simulink model "sampleModel1721"  (R2023a)
settings: Solver=VariableStepAuto  StartTime=0.0  StopTime=10.0  RelTol=1e-3
libraries: hdlsllib x3, simulink x1
settings Model: Creator=user1  LastModifiedBy=user1

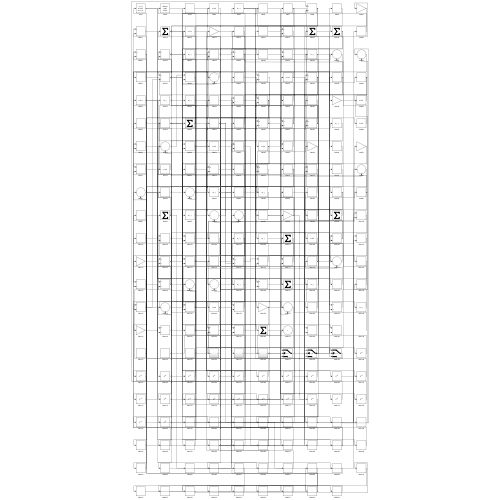
[thumbnail: Simulink's stored preview of the top-level diagram]
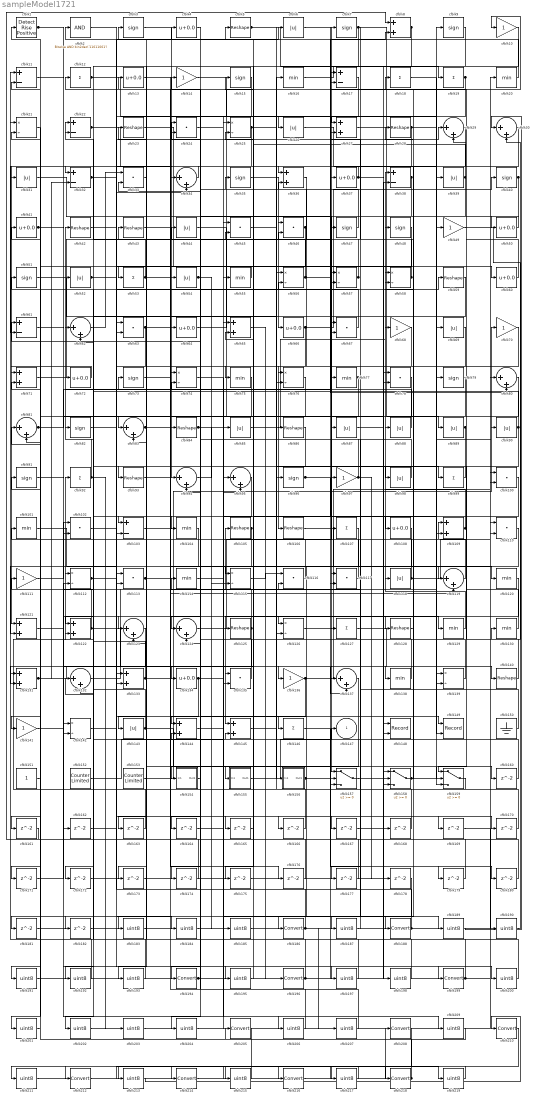
== system sampleModel1721 ==
  cfblk1 : hdlsllib/Logic and Bit Operations/Detect Rise Positive  vinit=0  OutDataTypeStr=boolean
  cfblk{10,14,49,68,70,97,111,136,141} (9 alike) : Gain
  cfblk{24,33,45..46,63,67,78,100,102,110,113,116..117,135} (14 alike) : DotProduct  OutDataTypeStr=Inherit: Inherit via internal rule
  cfblk{16,20,55,75,77,101,104,114,120,129..130,138} (12 alike) : MinMax
  cfblk{11,17,22,32,38,61,103} (7 alike) : Sum  Inputs=+-
  cfblk{5,23,28,42..43,59,84,86,93,105..106,125,128,140} (14 alike) : Reshape
  cfblk{12,18..19,53,92,99,107,127,146} (9 alike) : Sum  Inputs=+
  cfblk{4,13,37,41,50,60,64,66,72,108,134} (11 alike) : Bias  Bias=0.0  SaturateOnIntegerOverflow=off
  cfblk{8,27,36,65,71,109,121..122,131,133,144..145} (12 alike) : Sum
  cfblk{21,25,56..58,74,76,112,115,126,139,142} (12 alike) : Product  Inputs=*/  RndMeth=Zero  SaturateOnIntegerOverflow=on
  cfblk{6,26,31,39,44,52,54,69,85,87..90,98,118,143} (16 alike) : Abs  SaturateOnIntegerOverflow=off
  cfblk{29..30,34,62,80..81,83,94..95,119,123..124,132,137} (14 alike) : Sum  Inputs=|++
  cfblk148 : Record  FileSettingsInternal="{\"entries\":[{\"content\":{\"excelSettings\":{\"content\":{},\"type\":\"Streamout.ExcelSettings\"}},\"type\":\"Streamout.FileSettingStorage\",\"uuid\":\"\"}],\"packageUris\":[\"http:\\/\\/schema.mathworks.com\\/mf0\\/streamout_blocks\\/R2020a\"],\"version\":\"1.0\"}"  Layout=[1 1]  SignalsInternal="{\"entries\":[{\"content\":{\"signals\":[{\"content\":{\"blockPath\":[],\"dimensions\":[1],\"domain\":\"\",\"lineColor\":\"#a2142f\",\"plots\":[1],\"port\":1,\"signalID\":3280,\"signalName\":\"XY Graph:1\"},\"type\":\"RecordBlkView.Signal\",\"uuid\":\"\"},{\"content\":{\"blockPath\":[],\"dimensions\":[1],\"domain\":\"\",\"lineColor\":\"#139fff\",\"plots\":[1],\"port\":2,\"signalID\":3283,\"signalName\":\"XY Graph:2\"},\"type\":\"RecordBlkView.Signal\",\"uuid\":\"\"}]},\"type\":\"RecordBlkView.InputSignals\",\"uuid\":\"\"}],\"packageUris\":[\"http:\\/\\/schema.mathworks.com\\/mf0\\/streamout_blocks\\/R2020a\"],\"version\":\"1.0\"}"  VisualizationBindings="{\"xyplotplugin\":{\"info\":[{\"series\":[{\"bindingParametersList\":[{\"parameter\":\"X-Axis\",\"signalID\":3280,\"signalName\":\"XY Graph:1\"},{\"parameter\":\"Y-Axis\",\"signalID\":3283,\"signalName\":\"XY Graph:2\"}],\"seriesID\":52436}],\"subplotID\":1}]}}"  CompatibilityTag=XY  st=-1
  cfblk149 : Record  FileSettingsInternal="{\"entries\":[{\"content\":{\"excelSettings\":{\"content\":{},\"type\":\"Streamout.ExcelSettings\"}},\"type\":\"Streamout.FileSettingStorage\",\"uuid\":\"\"}],\"packageUris\":[\"http:\\/\\/schema.mathworks.com\\/mf0\\/streamout_blocks\\/R2020a\"],\"version\":\"1.0\"}"  Layout=[1 1]  SignalsInternal="{\"entries\":[{\"content\":{\"signals\":[{\"content\":{\"blockPath\":[],\"dimensions\":[1],\"domain\":\"\",\"lineColor\":\"#a2142f\",\"plots\":[1],\"port\":1,\"signalID\":3288,\"signalName\":\"XY Graph:1\"},\"type\":\"RecordBlkView.Signal\",\"uuid\":\"\"},{\"content\":{\"blockPath\":[],\"dimensions\":[1],\"domain\":\"\",\"lineColor\":\"#139fff\",\"plots\":[1],\"port\":2,\"signalID\":3291,\"signalName\":\"XY Graph:2\"},\"type\":\"RecordBlkView.Signal\",\"uuid\":\"\"}]},\"type\":\"RecordBlkView.InputSignals\",\"uuid\":\"\"}],\"packageUris\":[\"http:\\/\\/schema.mathworks.com\\/mf0\\/streamout_blocks\\/R2020a\"],\"version\":\"1.0\"}"  VisualizationBindings="{\"xyplotplugin\":{\"info\":[{\"series\":[{\"bindingParametersList\":[{\"parameter\":\"X-Axis\",\"signalID\":3288,\"signalName\":\"XY Graph:1\"},{\"parameter\":\"Y-Axis\",\"signalID\":3291,\"signalName\":\"XY Graph:2\"}],\"seriesID\":62969}],\"subplotID\":1}]}}"  CompatibilityTag=XY  st=-1
  cfblk{3,7,9,15,35,40,47..48,51,73,79,82,91,96} (14 alike) : Signum
  cfblk150 : Ground
  cfblk151 : Constant  SampleTime=-1
  cfblk152 : hdlsllib/Sources/Counter Limited  uplimit=7  tsamp=-1
  cfblk153 : hdlsllib/Sources/Counter Limited  uplimit=7  tsamp=-1
  cfblk154 : Subsystem
      settings: LibrarySourceBlock=|
      | hdlsllib/Ports &
      | Subsystems/Subsystem
  cfblk155 : Subsystem
      settings: LibrarySourceBlock=|
      | hdlsllib/Ports &
      | Subsystems/Subsystem
  cfblk156 : Subsystem
      settings: LibrarySourceBlock=|
      | hdlsllib/Ports &
      | Subsystems/Subsystem
  cfblk157 : Switch  SaturateOnIntegerOverflow=off  InputSameDT=off
  cfblk158 : Switch  SaturateOnIntegerOverflow=off  InputSameDT=off
  cfblk159 : Switch  SaturateOnIntegerOverflow=off  InputSameDT=off
  cfblk{160..182} (23 alike) : Delay  SampleTime=1
  cfblk{183..185,187,189..193,195,197..198,200..204,206..207,209,211,213,215,217,219} (25 alike) : DataTypeConversion  OutDataTypeStr=uint8  SaturateOnIntegerOverflow=off  RndMeth=Floor
  cfblk{186,188,194,196,199,205,208,210,212,214,216,218} (12 alike) : DataTypeConversion  SaturateOnIntegerOverflow=off  RndMeth=Floor
  cfblk2 : simulink/Logic and Bit Operations/Bitwise Operator  logicop=AND  UseBitMask=on  BitMask=bin2dec('11011001')  BitMaskRealWorld=Stored Integer
      settings: LibrarySourceBlock=|
      | hdlsllib/Logic and Bit
      | Operations/Bitwise
      | Operator
  cfblk147 : Outport  VectorParamsAs1DForOutWhenUnconnected=off
  wires:
  cfblk20/1 -> cfblk2/1
  cfblk156/1(Out1) -> cfblk58/1, cfblk180/1
  cfblk64/1 -> cfblk10/1
  cfblk94/1 -> cfblk85/1
  cfblk115/1 -> cfblk116/1
  cfblk62/1 -> cfblk33/1
  cfblk22/1 -> cfblk94/1, cfblk4/1
  cfblk125/1 -> cfblk105/1, cfblk131/2
  cfblk131/1 -> cfblk138/1, cfblk32/2
  cfblk7/1 -> cfblk89/1, cfblk182/1, cfblk187/1
  cfblk93/1 -> cfblk146/1
  cfblk8/1 -> cfblk143/1, cfblk83/2
  cfblk25/1 -> cfblk121/1, cfblk137/1, cfblk175/1
  cfblk52/1 -> cfblk148/2, cfblk166/1, cfblk167/1
  cfblk23/1 -> cfblk60/1
  cfblk107/1 -> cfblk186/1
  cfblk14/1 -> cfblk26/1
  cfblk145/1 -> cfblk16/1
  cfblk84/1 -> cfblk45/1, cfblk108/1
  cfblk159/1 -> cfblk92/1
  cfblk88/1 -> cfblk42/1
  cfblk153/1 -> cfblk79/1
  cfblk16/1 -> cfblk19/1
  cfblk40/1 -> cfblk66/1, cfblk50/1
  cfblk104/1 -> cfblk141/1
  cfblk129/1 -> cfblk38/1
  cfblk127/1 -> cfblk140/1
  cfblk85/1 -> cfblk68/1
  cfblk120/1 -> cfblk145/1
  cfblk114/1 -> cfblk25/1
  cfblk33/1 -> cfblk83/1
  cfblk71/1 -> cfblk7/1
  cfblk69/1 -> cfblk106/1
  cfblk59/1 -> cfblk122/1
  cfblk109/1 -> cfblk88/1, cfblk58/2
  cfblk44/1 -> cfblk148/1
  cfblk3/1 -> cfblk84/1
  cfblk124/1 -> cfblk37/1
  cfblk91/1 -> cfblk126/1
  cfblk11/1 -> cfblk199/1
  cfblk38/1 -> cfblk157/1, cfblk204/1
  cfblk66/1 -> cfblk9/1, cfblk75/1
  cfblk34/1 -> cfblk31/1
  cfblk30/1 -> cfblk188/1
  cfblk122/1 -> cfblk136/1, cfblk91/1
  cfblk141/1 -> cfblk116/2
  cfblk126/1 -> cfblk118/1
  cfblk82/1 -> cfblk44/1
  cfblk83/1 -> cfblk23/1, cfblk56/2, cfblk119/1
  cfblk106/1 -> cfblk120/1
  cfblk49/1 -> cfblk130/1
  cfblk28/1 -> cfblk139/1, cfblk61/2
  cfblk100/1 -> cfblk125/1
  cfblk103/1 -> cfblk70/1
  cfblk75/1 -> cfblk93/1
  cfblk43/1 -> cfblk64/1
  cfblk68/1 -> cfblk113/2
  cfblk132/1 -> cfblk39/1
  cfblk143/1 -> cfblk112/1, cfblk159/2, cfblk119/2
  cfblk108/1 -> cfblk126/2
  cfblk139/1 -> cfblk51/1
  cfblk5/1 -> cfblk158/3, cfblk99/1, cfblk117/1
  cfblk39/1 -> cfblk135/1, cfblk5/1, cfblk76/2
  cfblk98/1 -> cfblk24/1
  cfblk150/1 -> cfblk114/1
  cfblk18/1 -> cfblk69/1
  cfblk155/1(Out1) -> cfblk147/1
  cfblk111/1 -> cfblk102/1
  cfblk57/1 -> cfblk22/1, cfblk36/2
  cfblk128/1 -> cfblk18/1
  cfblk35/1 -> cfblk46/1
  cfblk113/1 -> cfblk129/1, cfblk17/2
  cfblk116/1 -> cfblk25/2
  cfblk6/1 -> cfblk67/1
  cfblk37/1 -> cfblk36/1, cfblk160/1
  cfblk86/1 -> cfblk103/1
  cfblk1/1 -> cfblk142/2, cfblk127/1
  cfblk89/1 -> cfblk132/2, cfblk193/1
  cfblk47/1 -> cfblk12/1
  cfblk90/1 -> cfblk159/1, cfblk62/2
  cfblk58/1 -> cfblk46/2, cfblk27/2
  cfblk92/1 -> cfblk62/1, cfblk203/1
  cfblk10/1 -> cfblk115/1
  cfblk70/1 -> cfblk124/1
  cfblk46/1 -> cfblk81/2, cfblk164/1
  cfblk154/1(Out1) -> cfblk94/2
  cfblk4/1 -> cfblk104/1
  cfblk32/1 -> cfblk6/1, cfblk34/1
  cfblk12/1 -> cfblk139/2, cfblk34/2
  cfblk63/1 -> cfblk54/1, cfblk155/1(In1), cfblk103/2
  cfblk119/1 -> cfblk43/1
  cfblk158/1 -> cfblk40/1, cfblk90/1, cfblk48/1, cfblk28/1
  cfblk53/1 -> cfblk22/2, cfblk159/3
  cfblk140/1 -> cfblk109/1
  cfblk51/1 -> cfblk156/1(In1)
  cfblk118/1 -> cfblk80/1, cfblk87/1
  cfblk45/1 -> cfblk96/1
  cfblk101/1 -> cfblk133/1
  cfblk97/1 -> cfblk14/1, cfblk178/1
  cfblk15/1 -> cfblk194/1
  cfblk2/1 -> cfblk57/1
  cfblk65/1 -> cfblk196/1
  cfblk67/1 -> cfblk13/1
  cfblk87/1 -> cfblk149/1
  cfblk142/1 -> cfblk59/1
  cfblk55/1 -> cfblk53/1
  cfblk144/1 -> cfblk97/1
  cfblk41/1 -> cfblk86/1, cfblk123/1
  cfblk134/1 -> cfblk144/1, cfblk189/1
  cfblk26/1 -> cfblk49/1
  cfblk130/1 -> cfblk17/1
  cfblk105/1 -> cfblk121/2, cfblk124/2
  cfblk36/1 -> cfblk76/1
  cfblk136/1 -> cfblk20/1, cfblk154/1(In1)
  cfblk56/1 -> cfblk35/1, cfblk80/2
  cfblk138/1 -> cfblk33/2
  cfblk50/1 -> cfblk47/1
  cfblk27/1 -> cfblk149/2
  cfblk31/1 -> cfblk67/2
  cfblk151/1 -> cfblk1/1
  cfblk133/1 -> cfblk82/1, cfblk169/1, cfblk170/1
  cfblk24/1 -> cfblk27/1
  cfblk117/1 -> cfblk101/1
  cfblk135/1 -> cfblk61/1
  cfblk79/1 -> cfblk128/1
  cfblk17/1 -> cfblk133/2
  cfblk54/1 -> cfblk115/2, cfblk185/1
  cfblk42/1 -> cfblk29/1
  cfblk110/1 -> cfblk134/1
  cfblk96/1 -> cfblk8/2, cfblk109/2
  cfblk60/1 -> cfblk29/2
  cfblk72/1 -> cfblk71/1
  cfblk81/1 -> cfblk102/2, cfblk77/1, cfblk137/2
  cfblk112/1 -> cfblk72/1, cfblk24/2
  cfblk9/1 -> cfblk32/1
  cfblk19/1 -> cfblk63/2, cfblk177/1
  cfblk77/1 -> cfblk171/1, cfblk172/1
  cfblk152/1 -> cfblk55/1
  cfblk99/1 -> cfblk98/1
  cfblk160/1 -> cfblk132/1
  cfblk76/1 -> cfblk161/1
  cfblk161/1 -> cfblk8/1
  cfblk121/1 -> cfblk162/1
  cfblk29/1 -> cfblk163/1
  cfblk163/1 -> cfblk122/2
  cfblk164/1 -> cfblk135/2
  cfblk73/1 -> cfblk165/1
  cfblk165/1 -> cfblk45/2
  cfblk166/1 -> cfblk81/1
  cfblk168/1 -> cfblk56/1
  cfblk170/1 -> cfblk123/2
  cfblk171/1 -> cfblk112/2
  cfblk172/1 -> cfblk157/2
  cfblk137/1 -> cfblk173/1
  cfblk173/1 -> cfblk38/2
  cfblk80/1 -> cfblk174/1
  cfblk174/1 -> cfblk131/1
  cfblk175/1 -> cfblk57/2
  cfblk13/1 -> cfblk176/1
  cfblk176/1 -> cfblk142/1
  cfblk177/1 -> cfblk71/2
  cfblk146/1 -> cfblk179/1
  cfblk179/1 -> cfblk158/2
  cfblk180/1 -> cfblk113/1
  cfblk48/1 -> cfblk181/1
  cfblk181/1 -> cfblk158/1
  cfblk182/1 -> cfblk157/3
  cfblk78/1 -> cfblk183/1
  cfblk183/1 -> cfblk100/1
  cfblk162/1 -> cfblk184/1
  cfblk184/1 -> cfblk78/1
  cfblk185/1 -> cfblk78/2
  cfblk186/1 -> cfblk63/1, cfblk207/1
  cfblk187/1 -> cfblk107/1
  cfblk188/1 -> cfblk100/2, cfblk145/2
  cfblk189/1 -> cfblk30/1
  cfblk169/1 -> cfblk190/1
  cfblk190/1 -> cfblk30/2
  cfblk21/1 -> cfblk191/1
  cfblk191/1 -> cfblk110/1
  cfblk123/1 -> cfblk192/1
  cfblk192/1 -> cfblk21/1
  cfblk193/1 -> cfblk21/2
  cfblk194/1 -> cfblk168/1, cfblk117/2, cfblk197/1
  cfblk102/1 -> cfblk195/1
  cfblk195/1 -> cfblk15/1
  cfblk196/1 -> cfblk52/1, cfblk73/1
  cfblk197/1 -> cfblk65/1
  cfblk167/1 -> cfblk198/1
  cfblk198/1 -> cfblk65/2
  cfblk199/1 -> cfblk144/2, cfblk3/1
  cfblk157/1 -> cfblk200/1
  cfblk200/1 -> cfblk11/1
  cfblk178/1 -> cfblk201/1
  cfblk201/1 -> cfblk11/2
  cfblk95/1 -> cfblk202/1
  cfblk202/1 -> cfblk110/2
  cfblk203/1 -> cfblk95/1
  cfblk204/1 -> cfblk95/2
  cfblk61/1 -> cfblk206/1
  cfblk206/1 -> cfblk74/1
  cfblk207/1 -> cfblk74/2
  cfblk74/1 -> cfblk209/1
  cfblk209/1 -> cfblk205/1
  cfblk205/1 -> cfblk211/1
  cfblk211/1 -> cfblk208/1
  cfblk208/1 -> cfblk213/1
  cfblk213/1 -> cfblk210/1
  cfblk210/1 -> cfblk215/1
  cfblk215/1 -> cfblk212/1
  cfblk216/1 -> cfblk218/1
  cfblk212/1 -> cfblk217/1
  cfblk217/1 -> cfblk214/1
  cfblk218/1 -> cfblk111/1, cfblk41/1
  cfblk214/1 -> cfblk219/1
  cfblk219/1 -> cfblk216/1

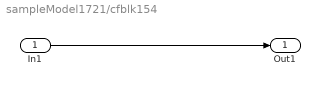
== system sampleModel1721/cfblk154 ==
  In1 : Inport
  Out1 : Outport
  wires:
  In1/1 -> Out1/1

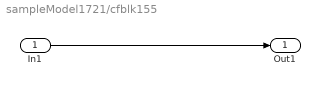
== system sampleModel1721/cfblk155 ==
  In1 : Inport
  Out1 : Outport
  wires:
  In1/1 -> Out1/1

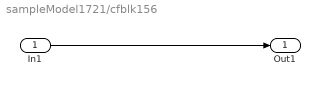
== system sampleModel1721/cfblk156 ==
  In1 : Inport
  Out1 : Outport
  wires:
  In1/1 -> Out1/1
